simulink model "progetto3Tenzo"  (Simulink 7.9)
settings: Solver=ode23s  StartTime=0.0  StopTime=80  RelTol=1e-3
values from neighbouring files (symbols this model uses):
  AMI = AK1    [AstaTenzoV3.m]
  AMin = [ ... (first row only)    [AstaTenzoV3.m]
  Aoss = AMin-V*ClocalMin    [AstaTenzoV3.m]
  BMI = BK1    [AstaTenzoV3.m]
  Bmod = [M BMin]    [AstaTenzoV3.m]
  Boss = [BMin-V*D V M-V*N]    [AstaTenzoV3.m]
  ClocalMin = [ ... (first row only)    [AstaTenzoV3.m]
  CMI = eye(q*mu)    [AstaTenzoV3.m]
  Coss = eye(n)    [AstaTenzoV3.m]
  D_phi = [1 325.437715018286 23852.1596168943 0]    [AstaTenzoV3.m]
  D_psi = [1 378.139322580724 35127.9961825618 0]    [AstaTenzoV3.m]
  D_theta = [1 325.437715018286 23852.1596168943 0]    [AstaTenzoV3.m]
  D_thrust = [1 963.786798861645 190423.384445206 0]    [AstaTenzoV3.m]
  DMI = zeros(q*mu,q)    [AstaTenzoV3.m]
  Dmod = [N D]    [AstaTenzoV3.m]
  Doss = zeros(size(Boss))    [AstaTenzoV3.m]
  F1 = F(:,size(AMin,1)+1:size(F,2))    [AstaTenzoV3.m]
  F2 = F(:,1:size(AMin,1))    [AstaTenzoV3.m]
  N_phi = [440.513056398418 26779.6272064186          272303.182447317 584729.91630594]    [AstaTenzoV3.m]
  N_psi = [59260.0621820611 3429565.45270113           27702908.9364068 53625940.9126871]    [AstaTenzoV3.m]
  N_theta = [440.513056398418 26779.6272064186          272303.182447317 584729.91630594]    [AstaTenzoV3.m]
  N_thrust = [682900.887332905 4668183.15145263]    [AstaTenzoV3.m]
  omega = 0.5    [AstaTenzoV3.m]
settings Model: Creator=danilo  LastModifiedBy=userk
settings DebuggingCC: FcnCallInpInsideContextMsg=Use local settings
settings GRTTargetCC: CombineOutputUpdateFcns=off  GRTInterface=on

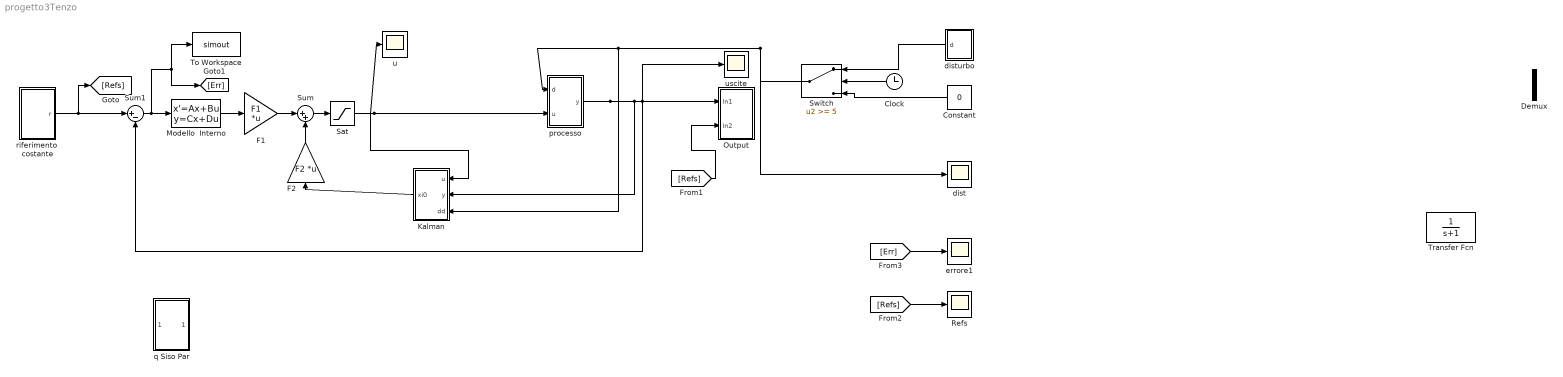
== system progetto3Tenzo ==
  Clock : Clock
  Constant : Constant  Value=0
  Demux : Demux  Outputs=2
  F1 : Gain  Gain=F1  Multiplication=Matrix(K*u) (u vector)
  F2 : Gain  Gain=F2  Multiplication=Matrix(K*u) (u vector)
  Kalman : Subsystem
  Modello  Interno : StateSpace  A=AMI  B=BMI  C=CMI  D=DMI
  Output : Subsystem
  Refs : Scope
  Sat : Saturate  UpperLimit=60  LowerLimit=-60
  Sum : Sum  Inputs=|++
  Sum1 : Sum  Inputs=|+-
  Switch : Switch  Threshold=5
  To Workspace : ToWorkspace  VariableName=simout  SampleTime=-1  SaveFormat=Structure
  Transfer Fcn : TransferFcn  Denominator=[1 1]
  dist : Scope
      settings: SaveName=ScopeData5
  disturbo : Subsystem
  errore1 : Scope
      settings: SaveName=ScopeData8
  processo : Subsystem
  "q Siso Par " : Subsystem
  riferimento  costante : Subsystem
  u : Scope
      settings: SaveName=ScopeData3
  uscite : Scope
      settings: SaveName=ScopeData2
  wires:
  riferimento  costante/1(r) -> Sum1/1, [Refs]
  processo/1(y) -> Kalman/2(y), Sum1/2, Output/1(In1), uscite/1
  Kalman/1(xi0) -> F2/1
  Modello  Interno/1 -> F1/1
  F2/1 -> Sum/2
  F1/1 -> Sum/1
  Sum/1 -> Sat/1
  Sum1/1 -> Modello  Interno/1, To Workspace/1, [Err]
  [Refs] -> Output/2(In2)
  [Refs] -> Refs/1
  [Err] -> errore1/1
  Clock/1 -> Switch/2
  Switch/1 -> dist/1, processo/1(d), Kalman/3(dd)
  disturbo/1(d) -> Switch/1
  Constant/1 -> Switch/3
  Sat/1 -> u/1, Kalman/1(u), processo/2(u)

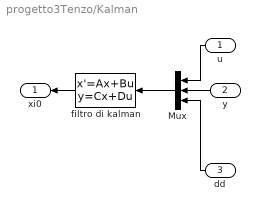
== system progetto3Tenzo/Kalman ==
  u : Inport
  y : Inport  Port=2
  dd : Inport  Port=3
  Mux : Mux  Inputs=[4 4 1]
  filtro di kalman : StateSpace  A=Aoss  B=Boss  C=Coss  D=Doss
  xi0 : Outport
  wires:
  Mux/1 -> filtro di kalman/1
  u/1 -> Mux/1
  filtro di kalman/1 -> xi0/1
  y/1 -> Mux/2
  dd/1 -> Mux/3

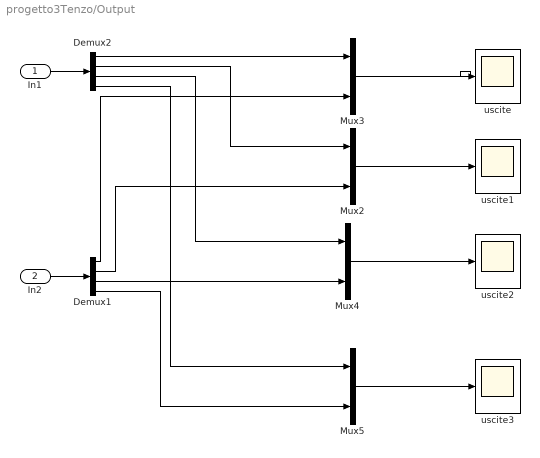
== system progetto3Tenzo/Output ==
  In1 : Inport
  In2 : Inport  Port=2
  Demux1 : Demux
  Demux2 : Demux
  Mux{2..5} (4 alike) : Mux  Inputs=2
  uscite{,1..3} (4 alike) : Scope
      uscite settings: TickLabels=on  YMin=-3.5  YMax=7
      uscite1 settings: TickLabels=on  TimeRange=30  YMin=0.75  YMax=4.25  SaveName=ScopeData4
      uscite2 settings: TickLabels=on  YMin=0.75  YMax=4.25  SaveName=ScopeData6
      uscite3 settings: TickLabels=on  YMin=0.75  YMax=4.25  SaveName=ScopeData7
  wires:
  Demux1/1 -> Mux3/2
  In2/1 -> Demux1/1
  In1/1 -> Demux2/1
  Mux3/1 -> uscite/1
  Demux2/1 -> Mux3/1
  Mux2/1 -> uscite1/1
  Demux2/2 -> Mux2/1
  Mux4/1 -> uscite2/1
  Demux2/3 -> Mux4/1
  Mux5/1 -> uscite3/1
  Demux2/4 -> Mux5/1
  Demux1/2 -> Mux2/2
  Demux1/3 -> Mux4/2
  Demux1/4 -> Mux5/2

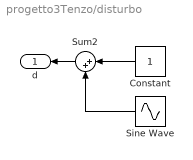
== system progetto3Tenzo/disturbo ==
  Constant : Constant
  Sine Wave : Sin  Amplitude=3  Frequency=omega  SampleTime=0
  Sum2 : Sum  Inputs=|++
  d : Outport
  wires:
  Sine Wave/1 -> Sum2/2
  Constant/1 -> Sum2/1
  Sum2/1 -> d/1

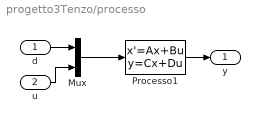
== system progetto3Tenzo/processo ==
  d : Inport
  u : Inport  Port=2
  Mux : Mux  Inputs=[1 4]
  Processo1 : StateSpace  A=AMin  B=Bmod  C=ClocalMin  D=Dmod
  y : Outport
  wires:
  Mux/1 -> Processo1/1
  d/1 -> Mux/1
  Processo1/1 -> y/1
  u/1 -> Mux/2

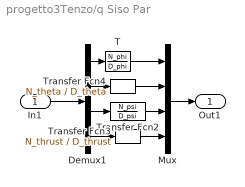
== system progetto3Tenzo/q Siso Par  ==
  In1 : Inport
  Demux1 : Demux
  Mux : Mux
  T : TransferFcn  Numerator=N_phi  Denominator=D_phi
  Transfer Fcn2 : TransferFcn  Numerator=N_psi  Denominator=D_psi
  Transfer Fcn3 : TransferFcn  Numerator=N_thrust  Denominator=D_thrust
  Transfer Fcn4 : TransferFcn  Numerator=N_theta  Denominator=D_theta
  Out1 : Outport
  wires:
  Mux/1 -> Out1/1
  In1/1 -> Demux1/1
  Transfer Fcn2/1 -> Mux/3
  Transfer Fcn4/1 -> Mux/2
  Demux1/2 -> Transfer Fcn4/1
  Transfer Fcn3/1 -> Mux/4
  T/1 -> Mux/1
  Demux1/4 -> Transfer Fcn3/1
  Demux1/3 -> Transfer Fcn2/1
  Demux1/1 -> T/1

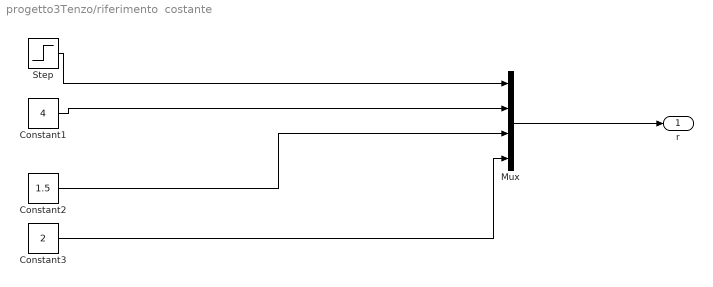
== system progetto3Tenzo/riferimento  costante ==
  Constant1 : Constant  Value=4
  Constant2 : Constant  Value=1.5
  Constant3 : Constant  Value=2
  Mux : Mux  Inputs=[1 1 1 1]
  Step : Step  Time=3  After=2.5  SampleTime=0
  r : Outport
  wires:
  Mux/1 -> r/1
  Step/1 -> Mux/1
  Constant1/1 -> Mux/2
  Constant2/1 -> Mux/3
  Constant3/1 -> Mux/4
